simulink model "KisaModel2012B"  (R2012b)
settings: Solver=ode45  StartTime=0.0  StopTime=15  RelTol=1e-3
libraries: fuzblock x1
settings Model: Creator=korisnik  LastModifiedBy=Aldin
settings DebuggingCC: FrameProcessingCompatibilityMsg=error
settings CodeAppCC: CustomSymbolStrType=$N$R$M_T
settings GRTTargetCC: CodeReplacementLibrary=C89/C90 (ANSI)

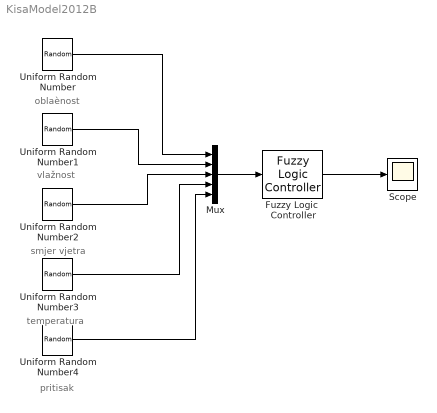
== system KisaModel2012B ==
  note: pritisak
  note: temperatura
  note: smjer vjetra
  note: vlažnost
  note: oblaènost
  Fuzzy Logic  Controller : fuzblock/Fuzzy Logic  Controller  FIS=zzz
  Mux : Mux  Inputs=5
  Scope : Scope
      settings: TimeRange=auto  LimitDataPoints=on  MaxDataPoints=5000  SaveToWorkspace=off  SaveName=ScopeData  YMin=-10  YMax=10  SampleTime=-1
  Uniform Random Number : UniformRandomNumber  Minimum=0  Maximum=10  SampleTime=0.1
  Uniform Random Number1 : UniformRandomNumber  Minimum=0  Maximum=100  SampleTime=0.1
  Uniform Random Number2 : UniformRandomNumber  Minimum=0  Maximum=360  SampleTime=0.1
  Uniform Random Number3 : UniformRandomNumber  Minimum=0  Maximum=40  SampleTime=0.1
  Uniform Random Number4 : UniformRandomNumber  Minimum=990  Maximum=1030  SampleTime=0.1
  wires:
  Uniform Random Number/1 -> Mux/1
  Uniform Random Number1/1 -> Mux/2
  Uniform Random Number2/1 -> Mux/3
  Uniform Random Number3/1 -> Mux/4
  Uniform Random Number4/1 -> Mux/5
  Mux/1 -> Fuzzy Logic  Controller/1
  Fuzzy Logic  Controller/1 -> Scope/1
